simulink model "PerformanceMetrics"  (R2024b)
settings: Solver=VariableStepAuto  StartTime=0.0  StopTime=10.0  RelTol=1e-3
settings Model: Creator=CArias  LastModifiedBy=CArias

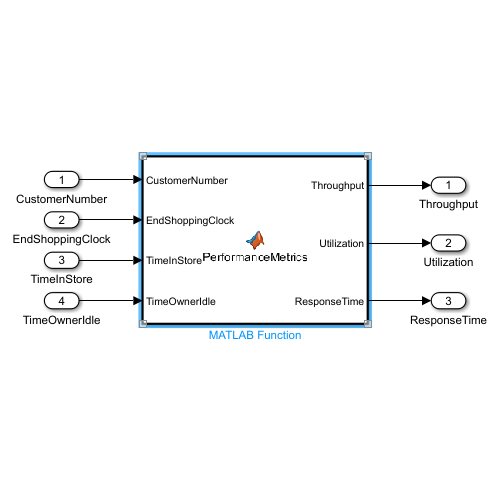
[thumbnail: Simulink's stored preview of the top-level diagram]
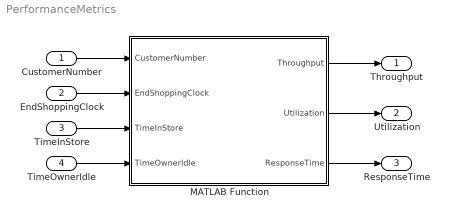
== system PerformanceMetrics ==
  CustomerNumber : Inport
  EndShoppingClock : Inport  Port=2
  TimeInStore : Inport  Port=3
  TimeOwnerIdle : Inport  Port=4
  MATLAB Function : MATLAB Function  TreatAsAtomicUnit=on
  Throughput : Outport
  Utilization : Outport  Port=2
  ResponseTime : Outport  Port=3
  wires:
  CustomerNumber/1 -> MATLAB Function/1(CustomerNumber)
  EndShoppingClock/1 -> MATLAB Function/2(EndShoppingClock)
  TimeInStore/1 -> MATLAB Function/3(TimeInStore)
  TimeOwnerIdle/1 -> MATLAB Function/4(TimeOwnerIdle)
  MATLAB Function/1(Throughput) -> Throughput/1
  MATLAB Function/2(Utilization) -> Utilization/1
  MATLAB Function/3(ResponseTime) -> ResponseTime/1

== matlab function PerformanceMetrics/MATLAB Function ==
  data: CustomerNumber input; Throughput output; EndShoppingClock input; TimeInStore input; TimeOwnerIdle input; Utilization output; ResponseTime output
function [Throughput, Utilization, ResponseTime] = PerformanceMetrics( ...
    CustomerNumber, EndShoppingClock, TimeInStore, TimeOwnerIdle)

    % Persistent variables to accumulate totals
    persistent TotalCompletionTime TotalOwnerBusyTime TotalStoreBusyTime NumberOfCompletions;
    
    if isempty(TotalCompletionTime)
        TotalCompletionTime = 0;
        TotalOwnerBusyTime = 0;
        TotalStoreBusyTime = 0;
        NumberOfCompletions = 0;
    end
    
    % Increment total completion time to reflect the latest EndShoppingClock
    TotalCompletionTime = EndShoppingClock;
    
    % Increment total store busy time with the time in store for the customer
    TotalStoreBusyTime = TotalStoreBusyTime + TimeInStore;
    
    % Increment total owner busy time by subtracting the idle time from the customer's total time
    OwnerBusyTime = TimeInStore - TimeOwnerIdle;
    TotalOwnerBusyTime = TotalOwnerBusyTime + max(0, OwnerBusyTime);
    
    % Increment the number of completed customers
    NumberOfCompletions = CustomerNumber;
    
    % Calculate observed time as the current total completion time
    ObservedTime = TotalCompletionTime;
    
    % Calculate Throughput: Number of completed jobs (customers) per observed time
    if ObservedTime > 0
        Throughput = NumberOfCompletions / ObservedTime;
    else
        Throughput = 0;
    end
    
    % Calculate Utilization: Owner busy time as a percentage of observed time
    if ObservedTime > 0
        Utilization = TotalOwnerBusyTime / ObservedTime;
    else
        Utilization = 0;
    end
    
    % Calculate ResponseTime: Average time in store per customer
    if NumberOfCompletions > 0
        ResponseTime = TotalStoreBusyTime / NumberOfCompletions;
    else
        ResponseTime = 0;
    end

end
